simulink model "DeadbeatSISO_WhiteNoise"  (R2016b)
settings: Solver=VariableStepAuto  StartTime=0.0  StopTime=10.0  RelTol=1e-3
values from neighbouring files (symbols this model uses):
  s = tf('s')    [Quantization_Analyzer.m]
  z = tf('z',1)    [Quantization_Analyzer.m]
libraries: cstblocks x2
settings Model: Creator=capn  LastModifiedBy=capn

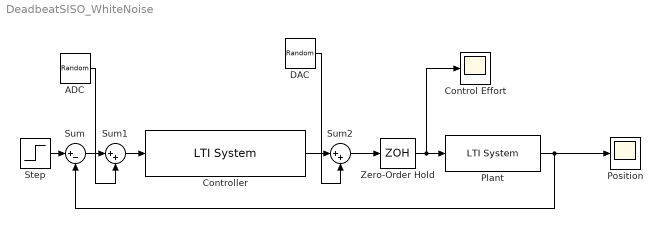
== system DeadbeatSISO_WhiteNoise ==
  ADC : RandomNumber  Variance=(4/1023)^2/12  SampleTime=0.1
  Control Effort : Scope
  Controller : cstblocks/LTI System  sys=(1.5820*z-0.5820)/(z+0.4180)  IC=[]
  DAC : RandomNumber  Variance=(10/256)^2/12  SampleTime=0.1
  Plant : cstblocks/LTI System  sys=1/s/(s+1)  IC=[]
  Position : Scope
  Step : Step  Time=0  SampleTime=0
  Sum : Sum  Inputs=|+-
  Sum1 : Sum  Inputs=|++
  Sum2 : Sum  Inputs=|++
  Zero-Order Hold : ZeroOrderHold  SampleTime=-1
  wires:
  Zero-Order Hold/1 -> Control Effort/1, Plant/1
  Step/1 -> Sum/1
  Plant/1 -> Position/1, Sum/2
  Sum/1 -> Sum1/1
  Sum1/1 -> Controller/1
  Controller/1 -> Sum2/1
  Sum2/1 -> Zero-Order Hold/1
  ADC/1 -> Sum1/2
  DAC/1 -> Sum2/2
